simulink library "TalariaParentModel"  (R2022b)
settings: Solver=VariableStepAuto  StartTime=0.0  StopTime=10.0  RelTol=1e-3
libraries: FeaturePath x1, StateVar x1, RTC x1, TuneVar x1
settings Model: Creator=kl13806  LastModifiedBy=kl13806
settings SolverCC: AlgebraicLoopSolver=TrustRegion
settings DebuggingCC: UnconnectedInputMsg=warning  UnconnectedOutputMsg=warning  UnconnectedLineMsg=warning  SFMachineParentedDataDiag=warning
settings ModelReferenceCC: EnableRefExpFcnMdlSchedulingChecks=on
settings RTWCC: DLArmComputeVersion=19.05

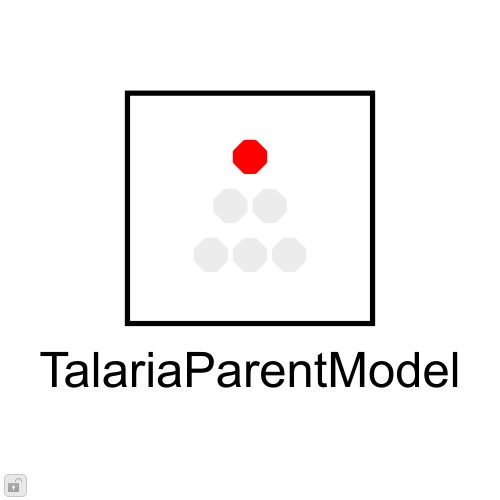
[thumbnail: Simulink's stored preview of the top-level diagram]
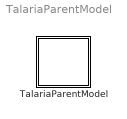
== system TalariaParentModel ==
  TalariaParentModel : Subsystem  TreatAsAtomicUnit=on  mask(Talaria Parent Model){TriggerInit=[]}
      mask prompts: TriggerInit "Hidden: dialog open, MoveFcn"
      mask help: This block ensures a top-level model that references other models will generate code for Talaria blocks even if the model itself does not otherwise contain any direct Talaria content.
      mask init:
      | [ok] = TalariaParentModelMask.DoInit(gcbh);
      settings: MoveFcn=TalariaParentModelMask.CB_TriggerInit(gcbh);
      mask Help: Place this block in a model's root diagram.
      mask Callback TriggerInit: TalariaParentModelMask.CB_TriggerInit(gcbh);
      mask DialogControl ErrorContainer Prompt: Error Messages
      mask Display:
      | % retrieve icon definition
      | [path,w,h] = TalariaParentModelMask.Icon();
      | 
      | % retrieve the block's pixel size
      | pos = get(gcbh,'position');
      | bw = pos(3) - pos(1);
      | bh = pos(4) - pos(2);
      | 
      | % draw centered icon
      | xAdj = bw/2 - w/2;
      | yAdj = bh/2 - h/2;
      | for i=1:length(path)
      |    patch(path(i).x+xAdj, path(i).y+yAdj, path(i).rgb);
      | end
      | 
      | % show the name or an X
      | if (exist('ok','var') && ok)
      |    patch(0,0,[1 1 1]);
      |    patch(bw,bh,[1 1 1]);
      | else
      |    tx=bw*0.03;
      |    ty=bh*0.03;
      |    patch([0 tx bw bw-tx], [ty 0 bh-ty bh], [1 0 0]);
      |    patch([0 bw-tx bw tx], [bh-ty 0 ty bh], [1 0 0]);
      | end

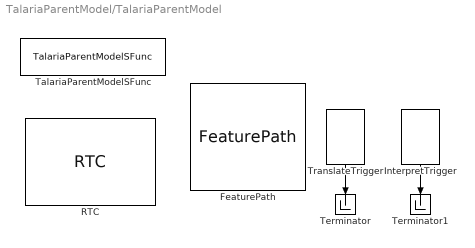
== system TalariaParentModel/TalariaParentModel ==
  FeaturePath : FeaturePath/FeaturePath  FeatureName=NoName  IsGroup=off  GroupNumber=-1  IsModule=off  TriggerInit=[130 179 245 286]
      settings: SourceProductName=Bose Talaria
  InterpretTrigger : StateVar/InterpretTrigger  TriggerInit=[341 205 379 260]
      settings: SourceProductName=Bose Talaria
  RTC : RTC/RTC  REQ_Priority=RTC_Mask.NormalPriority  RequestAtInit=off  EnableRequest=off  REQElemType1=uint32  REQElemWidth1=1  REQElemInitial1=[]  REQElemType2=uint32  REQElemWidth2=1  REQElemInitial2=[]  REQElemType3=uint32  REQElemWidth3=1  REQElemInitial3=[]  REQElemType4=uint32  REQElemWidth4=1  REQElemInitial4=[]  REQElemType5=uint32  REQElemWidth5=1  REQElemInitial5=[]  REQElemType6=uint32  REQElemWidth6=1  REQElemInitial6=[]  REQElemType7=uint32  REQElemWidth7=1  REQElemInitial7=[]  REQElemType8=uint32  REQElemWidth8=1  REQElemInitial8=[]  REQElemType9=uint32  REQElemWidth9=1  REQElemInitial9=[]  REQElemType10=uint32  REQElemWidth10=1  REQElemInitial10=[]  EnableResponse=off  EnableRSP_StatusIn=off  RSPElemType1=uint32  RSPElemWidth1=1  RSPElemType2=uint32  RSPElemWidth2=1  RSPElemType3=uint32  RSPElemWidth3=1  RSPElemType4=uint32  RSPElemWidth4=1  RSPElemType5=uint32  RSPElemWidth5=1  RSPElemType6=uint32  RSPElemWidth6=1  RSPElemType7=uint32  RSPElemWidth7=1  RSPElemType8=uint32  RSPElemWidth8=1  RSPElemType9=uint32  RSPElemWidth9=1  RSPElemType10=uint32  RSPElemWidth10=1  EnableNotification=off  EnableNTF_PrepTrig=off  NTFElemType1=uint32  NTFElemWidth1=1  NTFElemType2=uint32  NTFElemWidth2=1  NTFElemType3=uint32  NTFElemWidth3=1  NTFElemType4=uint32  NTFElemWidth4=1  NTFElemType5=uint32  NTFElemWidth5=1  NTFElemType6=uint32  NTFElemWidth6=1  NTFElemType7=uint32  NTFElemWidth7=1  NTFElemType8=uint32  NTFElemWidth8=1  NTFElemType9=uint32  NTFElemWidth9=1  NTFElemType10=uint32  NTFElemWidth10=1  MaskMessageName=..........
      settings: SourceProductName=Bose Talaria
  TalariaParentModelSFunc : M-S-Function  FunctionName=TalariaParentModelSFunc
  Terminator : Terminator
  Terminator1 : Terminator
  TranslateTrigger : TuneVar/TranslateTrigger  TriggerInit=[266 205 304 260]
      settings: SourceProductName=Bose Talaria
  wires:
  TranslateTrigger/1 -> Terminator/1
  InterpretTrigger/1 -> Terminator1/1
